simulink model "Beobachter_mit_I"  (R2019a)
settings: Solver=VariableStepAuto  StartTime=0.0  StopTime=10.0  RelTol=1e-3
values from neighbouring files (symbols this model uses):
  A = [0 1 0 0;m*g*l(M+m)/d 0 0 m*l*b/d;0 0 0 1;-g*m^2*l^2/d 0 0 -b*(I+m*l^2)/d]    [inv_pend.m]
  B = [0;-m*l/d;0;(I+m*l^2)/d]    [inv_pend.m]
  C = [0 0 1 0;1 0 0 0]    [inv_pend.m]
  K1 = KI(:,1:end-size(Cn,1))    [inv_pend.m]
  K2 = KI(:,end-size(Cn,1)+1:end)    [inv_pend.m]
  L = place(A',C',[-30 -31 -32 -33])'    [inv_pend.m]
settings Model: Creator=Naveen  LastModifiedBy=Naveen

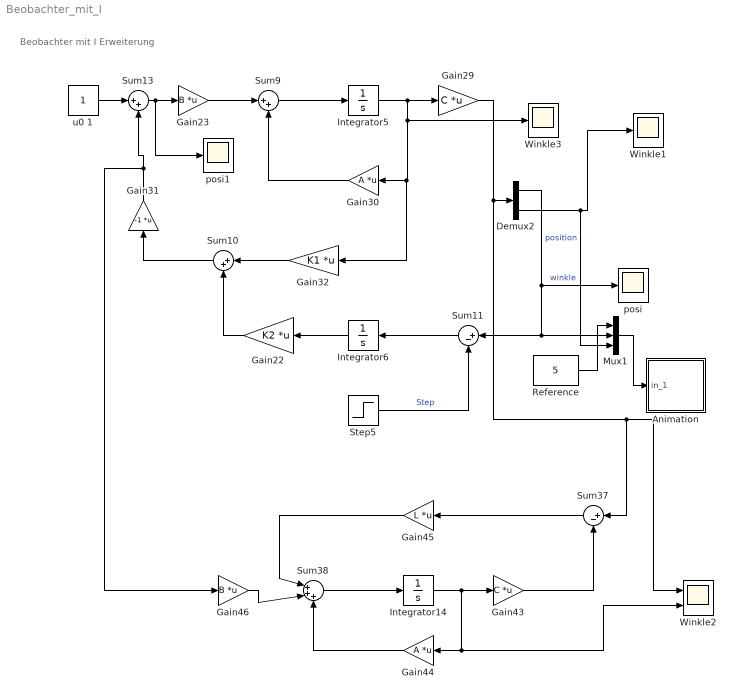
== system Beobachter_mit_I ==
  note: Beobachter mit I Erweiterung
  Animation : Subsystem  mask(Pendulum plot){RefBlock=Reference}
      mask prompts: RefBlock "DC reference signal block name:"
      mask help: Pendulum plot
      mask Help: Pendulum animation function using Handle graphics.
      mask Display: plot([-10 10],[0 0],[-2 -2 2 2],[0 1 1 0],[0 3],[1 5])
  Demux2 : Demux  Outputs=2
  Gain22 : Gain  Gain=K2  Multiplication=Matrix(K*u)
  Gain23 : Gain  Gain=B  Multiplication=Matrix(K*u)
  Gain29 : Gain  Gain=C  Multiplication=Matrix(K*u)
  Gain30 : Gain  Gain=A  Multiplication=Matrix(K*u)
  Gain31 : Gain  Gain=-1  Multiplication=Matrix(K*u)
  Gain32 : Gain  Gain=K1  Multiplication=Matrix(K*u)
  Gain43 : Gain  Gain=C  Multiplication=Matrix(K*u)
  Gain44 : Gain  Gain=A  Multiplication=Matrix(K*u)
  Gain45 : Gain  Gain=L  Multiplication=Matrix(K*u)
  Gain46 : Gain  Gain=B  Multiplication=Matrix(K*u)
  Integrator14 : Integrator  InitialCondition=0.1
  Integrator5 : Integrator
  Integrator6 : Integrator
  Mux1 : Mux  Inputs=3
  Reference : Constant  Value=5
  Step5 : Step  Time=0  After=5  SampleTime=0
  Sum10 : Sum  Inputs=|++
  Sum11 : Sum  Inputs=|+-
  Sum13 : Sum  Inputs=|++
  Sum37 : Sum  Inputs=|+-
  Sum38 : Sum  Inputs=|+++
  Sum9 : Sum  Inputs=|++
  Winkle1 : Scope
  Winkle2 : Scope  NumInputPorts=2
  Winkle3 : Scope
  posi : Scope
  posi1 : Scope
  u0 1 : Constant
  wires:
  Gain43/1 -> Sum37/2
  Sum38/1 -> Integrator14/1
  Gain29/1 -> Winkle2/1, Sum37/1, Demux2/1
  Gain45/1 -> Sum38/1
  Gain22/1 -> Sum10/2
  Sum10/1 -> Gain31/1
  Sum11/1 -> Integrator6/1
  Gain31/1 -> Gain46/1, Sum13/2
  Sum13/1 -> posi1/1, Gain23/1
  Sum9/1 -> Integrator5/1
  Gain30/1 -> Sum9/2
  Integrator5/1 -> Gain32/1, Gain30/1, Winkle3/1, Gain29/1
  Gain23/1 -> Sum9/1
  Integrator6/1 -> Gain22/1
  Sum37/1 -> Gain45/1
  Integrator14/1 -> Gain43/1, Gain44/1, Winkle2/2
  Gain46/1 -> Sum38/2
  Gain44/1 -> Sum38/3
  u0 1/1 -> Sum13/1
  Gain32/1 -> Sum10/1
  Step5/1 -> Sum11/2  "Step"
  Reference/1 -> Mux1/1
  Demux2/2 -> Mux1/3, Winkle1/1  "winkle"
  Mux1/1 -> Animation/1(in_1)
  Demux2/1 -> Mux1/2, Sum11/1, posi/1  "position"

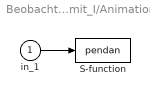
== system Beobachter_mit_I/Animation ==
  in_1 : Inport
  S-function : S-Function  FunctionName=pendan  Parameters=RefBlock  SFunctionDeploymentMode=off  EnableBusSupport=off
      settings: DeleteFcn=pendan([],[],[],'DeleteBlock');
  wires:
  in_1/1 -> S-function/1
